simulink model "EvenOddDetector"  (R2021a)
settings: Solver=VariableStepAuto  StartTime=0.0  StopTime=10.0  RelTol=1e-3
settings Model: Creator=NoteBook  LastModifiedBy=NoteBook

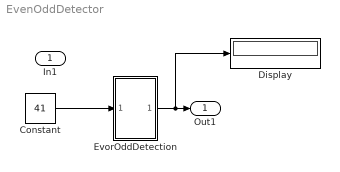
== system EvenOddDetector ==
  In1 : Inport
  Constant : Constant  Value=41
  Display : Display
  EvorOddDetection : Subsystem  TreatAsAtomicUnit=on
      settings: RTWFcnNameOpts=Use subsystem name  RTWFileNameOpts=Use subsystem name
  Out1 : Outport
  wires:
  EvorOddDetection/1(Out1) -> Display/1, Out1/1
  Constant/1 -> EvorOddDetection/1(In1)

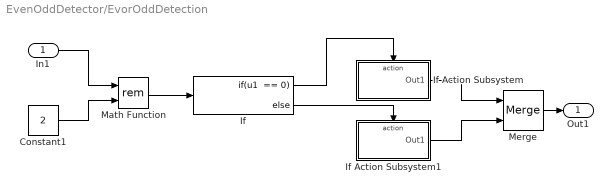
== system EvenOddDetector/EvorOddDetection ==
  In1 : Inport
  Constant1 : Constant  Value=2
  If : If  IfExpression="u1  == 0"
  If Action Subsystem : Subsystem  TreatAsAtomicUnit=on
  If Action Subsystem1 : Subsystem  TreatAsAtomicUnit=on
  Math Function : Math  Operator=rem  SaturateOnIntegerOverflow=on
  Merge : Merge
  Out1 : Outport
  wires:
  If/2 -> If Action Subsystem1/Action
  Constant1/1 -> Math Function/2
  Merge/1 -> Out1/1
  If Action Subsystem1/1(Out1) -> Merge/2
  If Action Subsystem/1(Out1) -> Merge/1
  If/1 -> If Action Subsystem/Action
  In1/1 -> Math Function/1
  Math Function/1 -> If/1

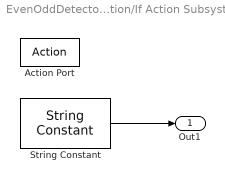
== system EvenOddDetector/EvorOddDetection/If Action Subsystem ==
  Action Port : ActionPort  ActionPortLabel="if(u1  == 0)"
  String Constant : StringConstant  String="\"Even\""
  Out1 : Outport
  wires:
  String Constant/1 -> Out1/1

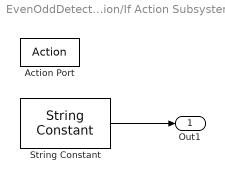
== system EvenOddDetector/EvorOddDetection/If Action Subsystem1 ==
  Action Port : ActionPort  ActionPortLabel=else
  String Constant : StringConstant  String="\"Odd\""
  Out1 : Outport
  wires:
  String Constant/1 -> Out1/1
